simulink model "Binary_FSK_Modulation"  (R2024a)
settings: Solver=VariableStepAuto  StartTime=0.0  StopTime=10.0  RelTol=1e-3
libraries: commrandsrc3 x1, commfilt2 x1
settings Model: Creator=alice  LastModifiedBy=alice

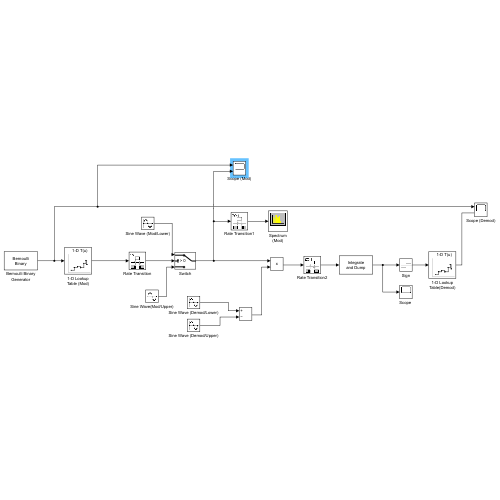
[thumbnail: Simulink's stored preview of the top-level diagram]
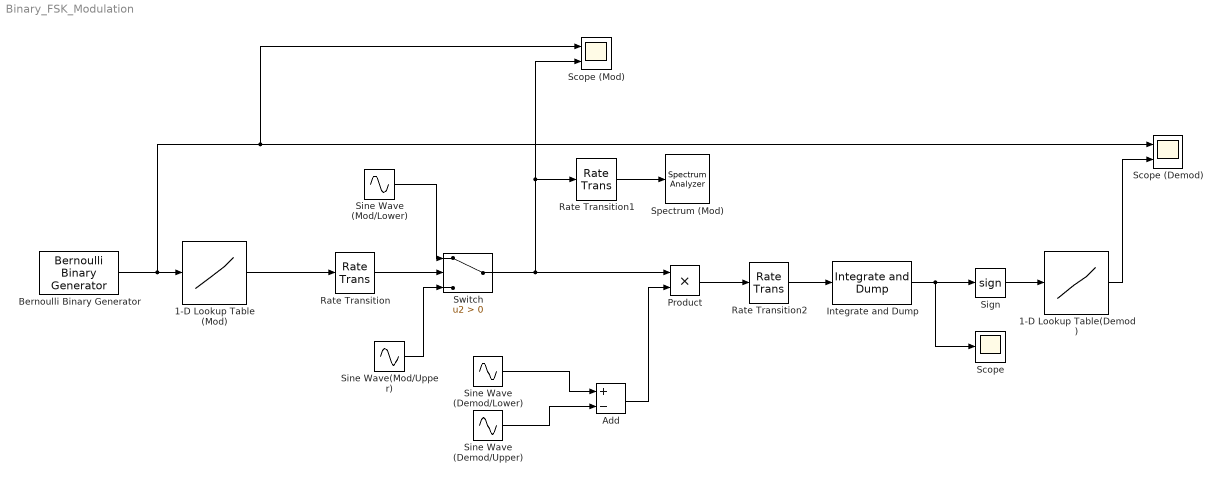
== system Binary_FSK_Modulation ==
  1-D Lookup Table (Mod) : Lookup_n-D  NumberOfTableDimensions=1  LookupTableObject=''  BreakpointsForDimension1=[0,1]  BreakpointsForDimension1FirstPoint=10  BreakpointsForDimension2FirstPoint=10  BreakpointsForDimension1Spacing=12  BreakpointsForDimension2Spacing=12  IndexSearchMethod=Evenly spaced points  Table=[-1,1]  InterpMethod=Flat  DiagnosticForOutOfRangeInput=Error  InternalRulePriority=Speed  RndMeth=Simplest
  1-D Lookup Table(Demod) : Lookup_n-D  NumberOfTableDimensions=1  LookupTableObject=''  BreakpointsForDimension1=[-1,0,1]  BreakpointsForDimension1FirstPoint=10  BreakpointsForDimension2FirstPoint=10  BreakpointsForDimension1Spacing=12  BreakpointsForDimension2Spacing=12  IndexSearchMethod=Evenly spaced points  Table=[0,0,1]  InterpMethod=Flat  DiagnosticForOutOfRangeInput=Error  InternalRulePriority=Speed  RndMeth=Simplest
  Add : Sum  Inputs=+-
  Bernoulli Binary Generator : commrandsrc3/Bernoulli Binary Generator  ProbabilityOfZero=0.5  SeedSource=Parameter  Seed=67  SampleTime=1e-3  SamplesPerFrame=1  OutputDataType=double  SimulateUsing=Interpreted execution
  Integrate and Dump : commfilt2/Integrate and Dump  obssamples=8  offsetsamples=0  nodump=off  roundingMode=Floor  overflowMode=off  outputDataTypeStr=Inherit: Same as accumulator  outputLastDataTypeStr=Inherit: Same as accumulator
  Product : Product
  Rate Transition : RateTransition  OutPortSampleTime=0.5e-4
  Rate Transition1 : RateTransition  OutPortSampleTime=0.5e-4
  Rate Transition2 : RateTransition  OutPortSampleTime=0.5e-4
  "Scope " : Scope
  Scope (Demod) : Scope  NumInputPorts=2
  Scope (Mod) : Scope  NumInputPorts=2
  Sign : Signum
  Sine Wave (Demod/Lower) : Sin  SineType=Sample based  Samples=4000  SampleTime=1e-7
  Sine Wave (Demod/Upper) : Sin  SineType=Sample based  Samples=2857  SampleTime=1e-7
  Sine Wave (Mod/Lower) : Sin  SineType=Sample based  Samples=4000  SampleTime=1e-7
  Sine Wave(Mod/Upper) : Sin  SineType=Sample based  Samples=2857  SampleTime=1e-7
  Spectrum (Mod) : SpectrumAnalyzer  WindowPosition=[1.000000,49.000000,1280.000000,729.000000,]  ScopeFrameLocation=window  YLimits=[-66.41140469,27.6368463]  SelectedToolstripTab=spectrumAnalyzerToolstrip.channelMeasurementsTab
  Switch : Switch  Criteria=u2 > Threshold  SaturateOnIntegerOverflow=off  InputSameDT=off
  wires:
  Bernoulli Binary Generator/1 -> Scope (Mod)/1, Scope (Demod)/1, 1-D Lookup Table (Mod)/1
  1-D Lookup Table (Mod)/1 -> Rate Transition/1
  Rate Transition/1 -> Switch/2
  Sine Wave(Mod/Upper)/1 -> Switch/3
  Sine Wave (Mod/Lower)/1 -> Switch/1
  Sine Wave (Demod/Lower)/1 -> Add/1
  Sine Wave (Demod/Upper)/1 -> Add/2
  Switch/1 -> Product/1, Rate Transition1/1, Scope (Mod)/2
  Rate Transition1/1 -> Spectrum (Mod)/1
  Add/1 -> Product/2
  Product/1 -> Rate Transition2/1
  Rate Transition2/1 -> Integrate and Dump/1
  Integrate and Dump/1 -> "Scope "/1, Sign/1
  Sign/1 -> 1-D Lookup Table(Demod)/1
  1-D Lookup Table(Demod)/1 -> Scope (Demod)/2
